simulink model "OL_Fre_Resp_Arduino"  (R2015a)
settings: Solver=FixedStepDiscrete  SolverMode=SingleTasking  StartTime=0.0  StopTime=inf  FixedStep=Ts  RelTol=1e-3
InitFcn:
  | Ts = 0.01;
  | rp = 2*pi/1336;
libraries: arduinolib x2, THLlib x2, simulink x1
settings Model: ExtModeTrigDuration=2  Creator=Carion  LastModifiedBy=SystemsUser
settings OptimizationCC: OptimizeModelRefInitCode=on  LifeSpan=1
settings DebuggingCC: UnderspecifiedInitializationDetection=Classic  MergeDetectMultiDrivingBlocksExec=none  StateNameClashWarn=warning
settings HardwareCC: ProdBitPerInt=16  ProdBitPerPointer=8  ProdIntDivRoundTo=Zero  ProdEndianess=LittleEndian  ProdWordSize=8  ProdHWDeviceType=Atmel->AVR
settings RTWCC: SystemTargetFile=realtime.tlc  GenerateMakefile=off  TemplateMakefile=realtime.tmf  Description=Run on Target Hardware  RTWVerbose=off
settings ERTTargetCC: CombineOutputUpdateFcns=off  ExtModeTransport=3  ExtModeMexFile=ext_serial_win32_comm  ExtModeMexArgs=0 1 9600  ERTSrcFileBannerTemplate=realtime_code_template.cgt  ERTHdrFileBannerTemplate=realtime_code_template.cgt  ERTDataSrcFileTemplate=realtime_code_template.cgt  ERTDataHdrFileTemplate=realtime_code_template.cgt  ERTCustomFileTemplate=realtime_file_process.tlc

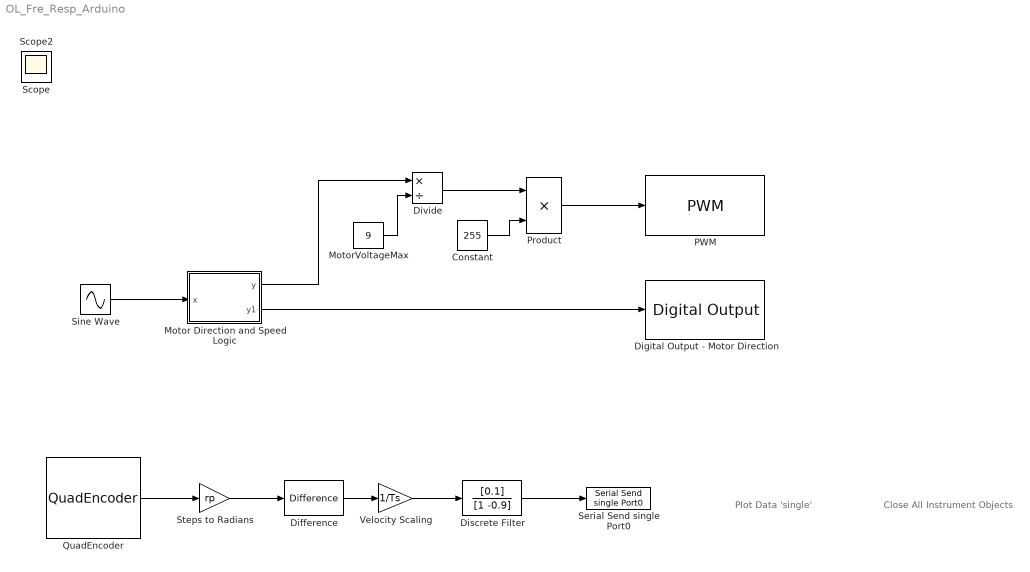
== system OL_Fre_Resp_Arduino ==
  note: Close All
      | Instrument Objects
  note: Plot Data
      | 'single'
  Constant : Constant  Value=255  SampleTime=Ts
  Difference : simulink/Discrete/Difference  ICPrevInput=0.0  InputProcessing=Inherited  OutMin=[]  OutMax=[]  OutDataType=fixdt(1, 16)  OutScaling=2^-10  DoSatur=off
  Digital Output - Motor Direction : arduinolib/Digital Output  pinNumber=4  blockPlatform=arduino
  Discrete Filter : DiscreteFilter  Numerator=[0.1]  Denominator=[1 -0.9]  SampleTime=Ts
  Divide : Product  Inputs=*/  SampleTime=Ts
  Motor Direction and Speed Logic : MATLAB Function  TreatAsAtomicUnit=on
  MotorVoltageMax : Constant  Value=9  SampleTime=Ts
  PWM : arduinolib/PWM  pinNumber=5  blockPlatform=arduino
  Product : Product  SampleTime=Ts
  QuadEncoder : THLlib/QuadEncoder
  Serial Send single Port0 : THLlib/Serial Send single Port0
  Sine Wave : Sin  Amplitude=4  Frequency=2*pi*1.5  SampleTime=Ts
  Steps to Radians : Gain  Gain=rp
  Velocity Scaling : Gain  Gain=1/Ts
  Scope : Scope
  Scope2 : Scope
      settings: SaveName=ScopeData2
  wires:
  Constant/1 -> Product/2
  Product/1 -> PWM/1
  MotorVoltageMax/1 -> Divide/2
  Divide/1 -> Product/1
  Motor Direction and Speed Logic/2(y1) -> Digital Output - Motor Direction/1
  Sine Wave/1 -> Motor Direction and Speed Logic/1(x)
  Motor Direction and Speed Logic/1(y) -> Divide/1
  QuadEncoder/1 -> Steps to Radians/1
  Steps to Radians/1 -> Difference/1
  Difference/1 -> Velocity Scaling/1
  Velocity Scaling/1 -> Discrete Filter/1
  Discrete Filter/1 -> Serial Send single Port0/1

== matlab function OL_Fre_Resp_Arduino/Motor Direction and Speed Logic ==
  data: x input; y output; y1 output
function [y,y1] = fcn(x)
%#codegen
if x>=0
    y=x;
    y1=0;
else
    y=-x;
    y1=1;
end
